simulink model "BulkMod_SMIA_SMIA_Sim"  (R2015a)
settings: Solver=ode4  StartTime=0.0  StopTime=tf  FixedStep=t_step  RelTol=1e-3
values from neighbouring files (symbols this model uses):
  Cp = 50e-6    (= 5e-05)    [BulkMod_SMIA_SMIA.m]    (also in Bulk_FL_PP_SE.m; Bulk_SM_PP_SE.m; Bulk_SM_SM_SE.m)
  Cpm = Cp * 1.1    (= 5.5e-05)    [BulkMod_SMIA_SMIA.m]
  DBm = DB * Ts / (2*L)    (= 0.04)    [BulkMod_SMIA_SMIA.m]    (also in Bulk_FL_PP_SE.m; Bulk_SM_PP_SE.m; Bulk_SM_SM_SE.m)
  Ks = 200 * Vi * lambda / ts    [BulkMod_SMIA_SMIA.m]    (also in Bulk_SM_PP_SE.m = 2 * Vi * (1 + lambda) / ts; Bulk_SM_SM_SE.m = Vi * (1 + lambda) / ts)
  L = 100e-6    (= 0.0001)    [BulkMod_SMIA_SMIA.m]    (also in Bulk_FL_PP_SE.m; Bulk_SM_PP_SE.m; Bulk_SM_SM_SE.m)
  lambda = 700    [BulkMod_SMIA_SMIA.m]    (also in Bulk_SM_PP_SE.m = 450; Bulk_SM_SM_SE.m)
  Lm = L * 1.1    (= 0.00011)    [BulkMod_SMIA_SMIA.m]
  phi = 0.001 * lambda^2    [BulkMod_SMIA_SMIA.m]    (also in Bulk_SM_PP_SE.m = 0.01 * lambda; Bulk_SM_SM_SE.m = 0.001 * lambda)
  R = 100    [BulkMod_SMIA_SMIA.m]    (also in Bulk_FL_PP_SE.m; Bulk_SM_PP_SE.m; Bulk_SM_SM_SE.m)
  Rm = R * 1.1    (= 110)    [BulkMod_SMIA_SMIA.m]
  Ts = 1e-5    (= 1e-05)    [BulkMod_SMIA_SMIA.m]    (also in Bulk_FL_PP_SE.m; Bulk_SM_PP_SE.m; Bulk_SM_SM_SE.m)
  Vi = 30    [BulkMod_SMIA_SMIA.m]    (also in Bulk_FL_PP_SE.m; Bulk_SM_PP_SE.m; Bulk_SM_SM_SE.m)
  Vim = Vi * 1.02    (= 30.6)    [BulkMod_SMIA_SMIA.m]
libraries: simulink x1
settings Model: Creator=Marcelo  LastModifiedBy=Marcelo

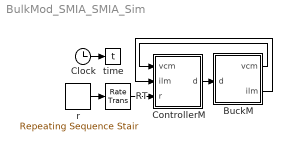
== system BulkMod_SMIA_SMIA_Sim ==
  BuckM : Subsystem
  Clock : Clock
  ControllerM : Subsystem
  RT : RateTransition  Integrity=off  Deterministic=off  X0=2
  r : simulink/Sources/Repeating Sequence Stair  OutValues=[2, 26, 14].'  tsamp=Tr  OutMin=[]  OutMax=[]  OutDataTypeStr=double  OutputDataTypeScalingMode=double  OutDataType=fixdt(0,8)  ConRadixGroup=Best Precision: Vector-wise  OutScaling=2^-12
  time : ToWorkspace  VariableName=t  SampleTime=-1
  wires:
  Clock/1 -> time/1
  BuckM/1(vcm) -> ControllerM/1(vcm)
  r/1 -> RT/1
  RT/1 -> ControllerM/3(r)
  ControllerM/1(d) -> BuckM/1(d)
  BuckM/2(ilm) -> ControllerM/2(ilm)

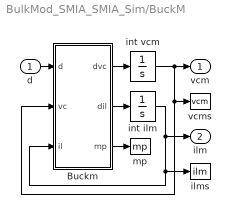
== system BulkMod_SMIA_SMIA_Sim/BuckM ==
  d : Inport
  Buckm : MATLAB Function  TreatAsAtomicUnit=on
  ilms : ToWorkspace  VariableName=ilm  SampleTime=-1
  int ilm : Integrator  LimitOutput=on  LowerSaturationLimit=0
  int vcm : Integrator  LimitOutput=on  LowerSaturationLimit=0
  mp : ToWorkspace  VariableName=mp  SampleTime=-1
  vcms : ToWorkspace  VariableName=vcm  SampleTime=-1
  vcm : Outport
  ilm : Outport  Port=2
  wires:
  int ilm/1 -> Buckm/3(il), ilms/1, ilm/1
  d/1 -> Buckm/1(d)
  int vcm/1 -> Buckm/2(vc), vcms/1, vcm/1
  Buckm/1(dvc) -> int vcm/1
  Buckm/2(dil) -> int ilm/1
  Buckm/3(mp) -> mp/1

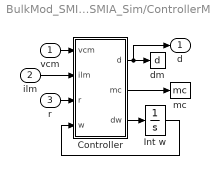
== system BulkMod_SMIA_SMIA_Sim/ControllerM ==
  vcm : Inport
  ilm : Inport  Port=2
  r : Inport  Port=3
  Controller : MATLAB Function  TreatAsAtomicUnit=on
  Int w : Integrator
  dm : ToWorkspace  VariableName=d  SampleTime=-1
  mc : ToWorkspace  VariableName=mc  SampleTime=-1
  d : Outport
  wires:
  Controller/1(d) -> d/1, dm/1
  vcm/1 -> Controller/1(vcm)
  r/1 -> Controller/3(r)
  Controller/2(mc) -> mc/1
  ilm/1 -> Controller/2(ilm)
  Controller/3(dw) -> Int w/1
  Int w/1 -> Controller/4(w)

== matlab function BulkMod_SMIA_SMIA_Sim/BuckM/Buckm ==
  data: d input; dvc output; vc input; il input; Vim parameter; Rm parameter; Lm parameter; Cpm parameter; dil output; Ts parameter; DBm parameter; mp output
function [dvc, dil, mp] = fcn(d, vc, il, Vim, Rm, Lm, Cpm, Ts, DBm)
dvc = (il - vc/Rm) / Cpm;
ilb = DBm * (Vim - vc);
if il < ilb % Nonlinear
    dil = Vim*d/Lm - 2*il*vc/(d*Ts*(Vim-vc));
    mp = 0;
else % Linear
    dil = Vim*d/Lm - vc/Lm;
    mp = 1;
end

== matlab function BulkMod_SMIA_SMIA_Sim/ControllerM/Controller ==
  data: vcm input; ilm input; r input; w input; R parameter; Cp parameter; L parameter; Vi parameter; Ts parameter; d output; DBm parameter; mc output size=1; lambda parameter; phi parameter; Ks parameter; dw output
function [d, mc, dw] = fcn(vcm, ilm, r, w, R, Cp, L, Vi, Ts, DBm, lambda, phi, Ks)
ilb = DBm * (Vi - vcm); % Conduction Mode Boundary
dvcm = (ilm - vcm/R) / Cp;
dw = vcm - r;
% Sliding Surface
s = dvcm + 2 * lambda * dw + lambda^2 * w;
% Slinding-Mode Integral Action Controller
sat_s = min(1, max(-1, s/phi));
v = - 2 * lambda * dvcm - lambda^2 * dw - Ks * sat_s;
if ilm < ilb %%%   NONLINEAR   %%%
    % Controller - Input-Output Linearization
    a = L * ((ilm - vcm/R)/(R*Cp) + Cp*v) / (2*Vi);
    b = 2 * ilm * vcm * L / (Vi * Ts * (Vi - vcm));
    d = a + sqrt(a^2 + b);
    mc = 0;
else         %%%   LINEAR      %%%
    % Controller - Pole Placement with Tracking
    d = (L * (Cp*v + (ilm - vcm/R) / (R*Cp)) + vcm) / Vi;
    mc = 1;
end

if d > 1
    d = 1;
elseif d < 1e-10
    d = 1e-10;
end
